simulink model "Base_Model_three_drones"  (R2025b)
settings: Solver=FixedStepDiscrete  StartTime=0.0  StopTime=10.0  FixedStep=0.01  RelTol=1e-3
values from neighbouring files (symbols this model uses):
  Attachment_Point_Vectors : value not decoded    [Base_Model.sldd]
  Cable_Damping = 0.1    [Base_Model.sldd]
  Cable_Resting_Length = 0.8    [Base_Model.sldd]
  Cable_Stiffness = 500.0    [Base_Model.sldd]
  Carrier_Mass = 0.01    [Base_Model.sldd]
  g = 9.81    [Base_Model.sldd]
  Kdc = 0.001    [Base_Model.sldd]
  Kpc = 10.0    [Base_Model.sldd]
  Load_Damping_Coef = 1.0    [Base_Model.sldd]
  Load_Inertia_Matrix : value not decoded    [Base_Model.sldd]
  Load_Mass = 0.7    [Base_Model.sldd]
undefined symbols (not defined in the file or in its folder): DiscIntNeverNeededParam
libraries: RotorSuite_lib x7, matrix_library x1, aerolibutil x1
settings Model: DataDictionary=Base_Model.sldd  Creator=lenovo  LastModifiedBy=lenovo

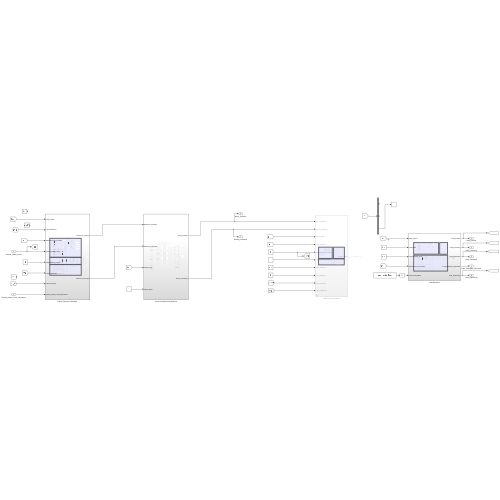
[thumbnail: Simulink's stored preview of the top-level diagram]
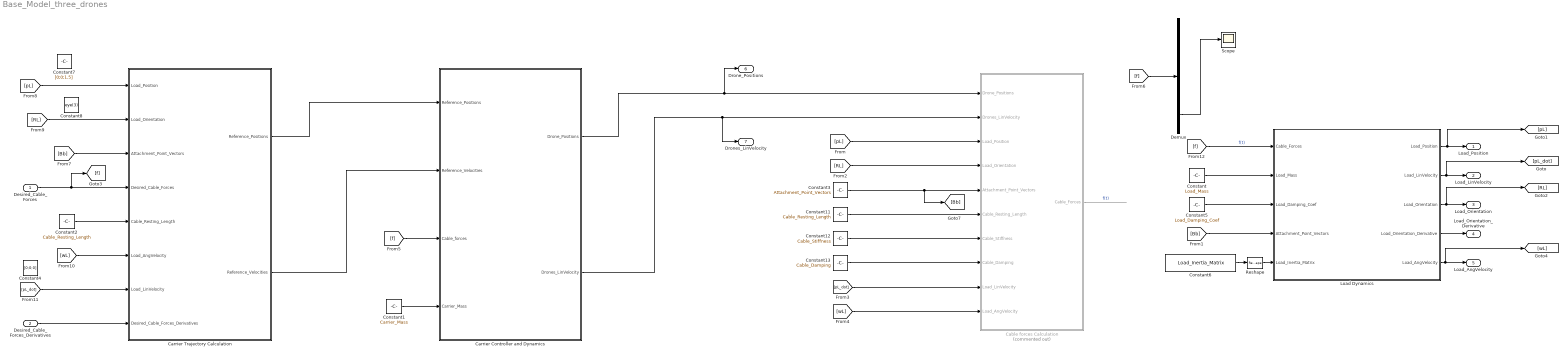
== system Base_Model_three_drones ==
  Desired_Cable_Forces : Inport
  Desired_Cable_Forces_Derivatives : Inport  Port=2
  Cable forces Calculation : Subsystem  Commented=on
  Carrier Controller and Dynamics : Subsystem
  "Carrier Trajectory Calculation " : Subsystem
  Constant : Constant  Value=Load_Mass
  Constant1 : Constant  Value=Carrier_Mass
  Constant11 : Constant  Value=Cable_Resting_Length
  Constant12 : Constant  Value=Cable_Stiffness
  Constant13 : Constant  Value=Cable_Damping
  Constant2 : Constant  Value=Cable_Resting_Length
  Constant3 : Constant  Value=Attachment_Point_Vectors
  Constant4 : Constant  Value=[0;0;0]
  Constant5 : Constant  Value=Load_Damping_Coef
  Constant6 : Constant  Value=Load_Inertia_Matrix
  Constant7 : Constant  Value=[0;0;1.5]
  Constant8 : Constant  Value=eye(3)
  Demux : Demux  Outputs=[3, 3, 3]
  Load Dynamics : Subsystem
  Reshape : Reshape  OutputDimensionality=Customize  OutputDimensions=[3,3]
  Scope : Scope
      settings: ActiveDisplayYMinimum=-1.9150350713046473E+13  ActiveDisplayYMaximum=2.47705516980144E+13
  Load_Position : Outport
  Load_LinVelocity : Outport  Port=2
  Load_Orientation : Outport  Port=3
  Load_Orientation_Derivative : Outport  Port=4
  Load_AngVelocity : Outport  Port=5
  Drone_Positions : Outport  Port=6
  Drones_LinVelocity : Outport  Port=7
  wires:
  Constant/1 -> Load Dynamics/2(Load_Mass)
  Constant5/1 -> Load Dynamics/3(Load_Damping_Coef)
  Constant6/1 -> Reshape/1
  Load Dynamics/2(Load_LinVelocity) -> [pL_dot], Load_LinVelocity/1
  Load Dynamics/1(Load_Position) -> [pL], Load_Position/1
  Load Dynamics/3(Load_Orientation) -> [RL], Load_Orientation/1
  Load Dynamics/5(Load_AngVelocity) -> [wL], Load_AngVelocity/1
  Cable forces Calculation/1(Cable_Forces) -> ?  "f(t)"
  [pL] -> Cable forces Calculation/3(Load_Position)
  [RL] -> Cable forces Calculation/4(Load_Orientation)
  Constant11/1 -> Cable forces Calculation/6(Cable_Resting_Length)
  [pL_dot] -> Cable forces Calculation/9(Load_LinVelocity)
  [wL] -> Cable forces Calculation/10(Load_AngVelocity)
  Constant12/1 -> Cable forces Calculation/7(Cable_Stiffness)
  Constant13/1 -> Cable forces Calculation/8(Cable_Damping)
  [Bb] -> Load Dynamics/4(Attachment_Point_Vectors)
  Carrier Controller and Dynamics/2(Drones_LinVelocity) -> Drones_LinVelocity/1, Cable forces Calculation/2(Drones_LinVelocity)
  [f] -> Carrier Controller and Dynamics/3(Cable_forces)
  Constant1/1 -> Carrier Controller and Dynamics/4(Carrier_Mass)
  "Carrier Trajectory Calculation "/1(Reference_Positions) -> Carrier Controller and Dynamics/1(Reference_Positions)
  Desired_Cable_Forces/1 -> [f], "Carrier Trajectory Calculation "/4(Desired_Cable_Forces)
  "Carrier Trajectory Calculation "/2(Reference_Velocities) -> Carrier Controller and Dynamics/2(Reference_Velocities)
  [Bb] -> "Carrier Trajectory Calculation "/3(Attachment_Point_Vectors)
  Constant2/1 -> "Carrier Trajectory Calculation "/5(Cable_Resting_Length)
  [wL] -> "Carrier Trajectory Calculation "/6(Load_AngVelocity)
  Desired_Cable_Forces_Derivatives/1 -> "Carrier Trajectory Calculation "/8(Desired_Cable_Forces_Derivatives)
  Load Dynamics/4(Load_Orientation_Derivative) -> Load_Orientation_Derivative/1
  Constant3/1 -> [Bb], Cable forces Calculation/5(Attachment_Point_Vectors)
  Reshape/1 -> Load Dynamics/5(Load_Inertia_Matrix)
  Demux/3 -> Scope/1
  [pL] -> "Carrier Trajectory Calculation "/1(Load_Position)
  [pL_dot] -> "Carrier Trajectory Calculation "/7(Load_LinVelocity)
  [f] -> Load Dynamics/1(Cable_Forces)  "f(t)"
  [f] -> Demux/1
  Carrier Controller and Dynamics/1(Drone_Positions) -> Drone_Positions/1, Cable forces Calculation/1(Drone_Positions)
  [RL] -> "Carrier Trajectory Calculation "/2(Load_Orientation)

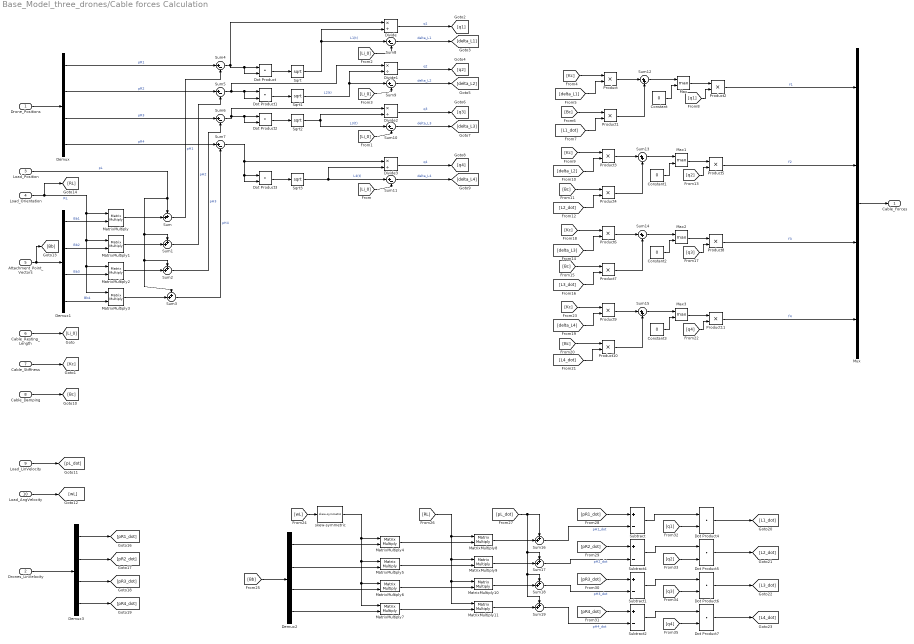
== system Base_Model_three_drones/Cable forces Calculation ==
  Drone_Positions : Inport
  Drones_LinVelocity : Inport  Port=2
  Load_Position : Inport  Port=3
  Load_Orientation : Inport  Port=4
  Attachment_Point_Vectors : Inport  Port=5
  Cable_Resting_Length : Inport  Port=6
  Cable_Stiffness : Inport  Port=7
  Cable_Damping : Inport  Port=8
  Load_LinVelocity : Inport  Port=9
  Load_AngVelocity : Inport  Port=10
  Constant{,1..3} (4 alike) : Constant  Value=0
  Demux : Demux
  Demux1 : Demux  Outputs=[3, 3, 3, 3]
  Demux2 : Demux
  Demux3 : Demux
  Divide{,1..3} (4 alike) : Product  Inputs=*/
  Dot Product{,1..7} (8 alike) : DotProduct  OutDataTypeStr=Inherit: Inherit via internal rule
  MatrixMultiply{,1..11} (12 alike) : Product  Multiplication=Matrix(*)
  Max{,1..3} (4 alike) : MinMax  Function=max  Inputs=2
  Mux : Mux
  Product{,1..11} (12 alike) : Product
  Sqrt{,1..3} (4 alike) : Sqrt
  Subtract{,1..2,4} (4 alike) : Sum  Inputs=+-
  Sum{,1..3,16..19} (8 alike) : Sum  Inputs=++|
  Sum{4..11} (8 alike) : Sum  Inputs=|+-
  Sum{12..15} (4 alike) : Sum  Inputs=|++
  skew-symmetric : RotorSuite_lib/Utils/skew-symmetric
  Cable_Forces : Outport
  wires:
  Mux/1 -> Cable_Forces/1
  Drone_Positions/1 -> Demux/1
  Attachment_Point_Vectors/1 -> Demux1/1, [Bb]
  Demux1/1 -> MatrixMultiply/2  "Bb1"
  Load_Orientation/1 -> [RL], MatrixMultiply3/1, MatrixMultiply2/1, MatrixMultiply1/1, MatrixMultiply/1  "RL"
  Demux1/2 -> MatrixMultiply1/2  "Bb2"
  Demux1/3 -> MatrixMultiply2/2  "Bb3"
  Demux1/4 -> MatrixMultiply3/2  "Bb4"
  MatrixMultiply/1 -> Sum/2
  Load_Position/1 -> Sum1/1, Sum2/1, Sum3/1, Sum/1  "pL"
  MatrixMultiply1/1 -> Sum1/2
  MatrixMultiply2/1 -> Sum2/2
  MatrixMultiply3/1 -> Sum3/2
  Demux/1 -> Sum4/1  "pR1"
  Demux/2 -> Sum5/1  "pR2"
  Demux/3 -> Sum6/1  "pR3"
  Demux/4 -> Sum7/1  "pR4"
  Sum/1 -> Sum4/2  "pH1"
  Sum1/1 -> Sum5/2  "pH2"
  Sum2/1 -> Sum6/2  "pH3"
  Sum3/1 -> Sum7/2  "pH4"
  Sum4/1 -> Dot Product/2, Dot Product/1, Divide/1
  Dot Product/1 -> Sqrt/1
  Dot Product1/1 -> Sqrt1/1
  Dot Product2/1 -> Sqrt2/1
  Dot Product3/1 -> Sqrt3/1
  Sqrt/1 -> Divide/2, Sum8/1  "L1(t)"
  Sqrt1/1 -> Sum9/1, Divide1/2  "L2(t)"
  Sum5/1 -> Dot Product1/2, Dot Product1/1, Divide1/1
  Sqrt2/1 -> Sum10/1, Divide2/2  "L3(t)"
  Sum6/1 -> Divide2/1, Dot Product2/2, Dot Product2/1
  Sqrt3/1 -> Divide3/2, Sum11/1  "L4(t)"
  Sum7/1 -> Divide3/1, Dot Product3/2, Dot Product3/1
  Cable_Resting_Length/1 -> [Li_0]
  Cable_Stiffness/1 -> [Kc]
  [Li_0] -> Sum11/2
  [Li_0] -> Sum10/2
  [Li_0] -> Sum8/2
  [Li_0] -> Sum9/2
  Divide/1 -> [q1]  "q1"
  Divide1/1 -> [q2]  "q2"
  Divide2/1 -> [q3]  "q3"
  Divide3/1 -> [q4]  "q4"
  Sum8/1 -> [delta_L1]  "delta_L1"
  Sum9/1 -> [delta_L2]  "delta_L2"
  Sum10/1 -> [delta_L3]  "delta_L3"
  Sum11/1 -> [delta_L4]  "delta_L4"
  [Kc] -> Product/1
  [delta_L1] -> Product/2
  Cable_Damping/1 -> [Bc]
  [L1_dot] -> Product1/2
  [Bc] -> Product1/1
  Product/1 -> Sum12/1
  Product1/1 -> Sum12/2
  Sum12/1 -> Max/1
  Constant/1 -> Max/2
  Max/1 -> Product2/1
  [q1] -> Product2/2
  Product2/1 -> Mux/1  "f1"
  [q2] -> Product5/2
  Max1/1 -> Product5/1
  Constant1/1 -> Max1/2
  Sum13/1 -> Max1/1
  Product4/1 -> Sum13/2
  Product3/1 -> Sum13/1
  [Bc] -> Product4/1
  [L2_dot] -> Product4/2
  [delta_L2] -> Product3/2
  [Kc] -> Product3/1
  Product5/1 -> Mux/2  "f2"
  [Kc] -> Product6/1
  [delta_L3] -> Product6/2
  [L3_dot] -> Product7/2
  [Bc] -> Product7/1
  Product6/1 -> Sum14/1
  Product7/1 -> Sum14/2
  Sum14/1 -> Max2/1
  Constant2/1 -> Max2/2
  Max2/1 -> Product8/1
  [q3] -> Product8/2
  Product8/1 -> Mux/3  "f3"
  [q4] -> Product11/2
  Max3/1 -> Product11/1
  Constant3/1 -> Max3/2
  Sum15/1 -> Max3/1
  Product10/1 -> Sum15/2
  Product9/1 -> Sum15/1
  [Bc] -> Product10/1
  [L4_dot] -> Product10/2
  [delta_L4] -> Product9/2
  [Kc] -> Product9/1
  Product11/1 -> Mux/4  "f4"
  Load_LinVelocity/1 -> [pL_dot]
  Load_AngVelocity/1 -> [wL]
  [Bb] -> Demux2/1
  [wL] -> skew-symmetric/1
  Demux2/1 -> MatrixMultiply4/2
  Demux2/2 -> MatrixMultiply5/2
  Demux2/3 -> MatrixMultiply6/2
  Demux2/4 -> MatrixMultiply7/2
  skew-symmetric/1 -> MatrixMultiply5/1, MatrixMultiply6/1, MatrixMultiply7/1, MatrixMultiply4/1
  MatrixMultiply4/1 -> MatrixMultiply8/2
  MatrixMultiply5/1 -> MatrixMultiply9/2
  MatrixMultiply6/1 -> MatrixMultiply10/2
  MatrixMultiply7/1 -> MatrixMultiply11/2
  [RL] -> MatrixMultiply11/1, MatrixMultiply10/1, MatrixMultiply9/1, MatrixMultiply8/1
  MatrixMultiply8/1 -> Sum16/2
  MatrixMultiply9/1 -> Sum17/2
  MatrixMultiply10/1 -> Sum18/2
  MatrixMultiply11/1 -> Sum19/2
  [pL_dot] -> Sum16/1, Sum19/1, Sum18/1, Sum17/1
  Drones_LinVelocity/1 -> Demux3/1
  Demux3/1 -> [pR1_dot]
  Demux3/2 -> [pR2_dot]
  Demux3/3 -> [pR3_dot]
  Demux3/4 -> [pR4_dot]
  Sum16/1 -> Subtract/2  "pH1_dot"
  [pR1_dot] -> Subtract/1
  [pR2_dot] -> Subtract4/1
  Sum17/1 -> Subtract4/2  "pH2_dot"
  [pR3_dot] -> Subtract1/1
  Sum18/1 -> Subtract1/2  "pH3_dot"
  Sum19/1 -> Subtract2/2  "pH4_dot"
  [pR4_dot] -> Subtract2/1
  Subtract/1 -> Dot Product4/1
  [q1] -> Dot Product4/2
  Subtract4/1 -> Dot Product5/1
  Subtract1/1 -> Dot Product6/1
  Subtract2/1 -> Dot Product7/1
  [q2] -> Dot Product5/2
  [q3] -> Dot Product6/2
  [q4] -> Dot Product7/2
  Dot Product4/1 -> [L1_dot]
  Dot Product5/1 -> [L2_dot]
  Dot Product6/1 -> [L3_dot]
  Dot Product7/1 -> [L4_dot]

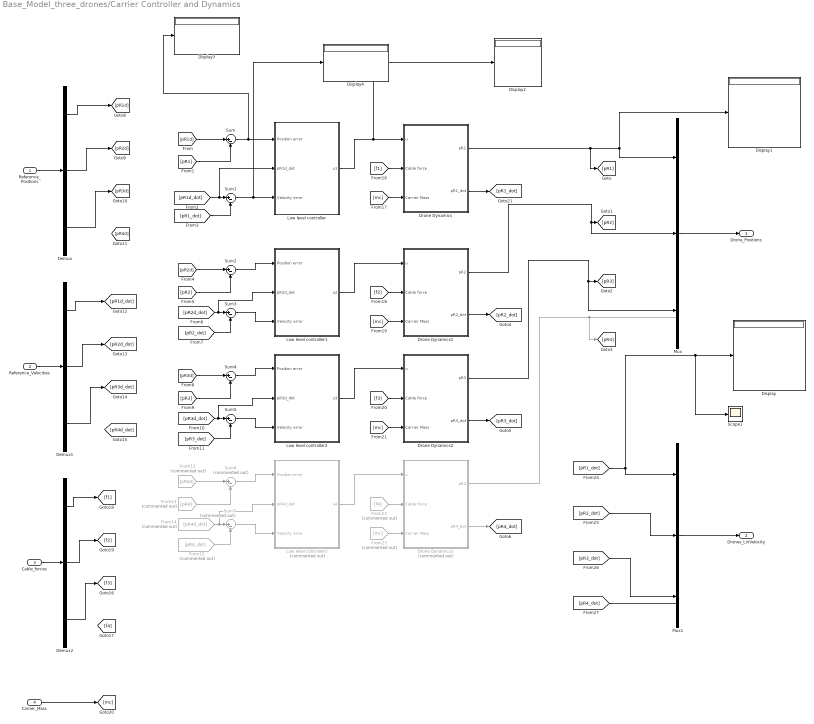
== system Base_Model_three_drones/Carrier Controller and Dynamics ==
  Reference_Positions : Inport
  Reference_Velocities : Inport  Port=2
  Cable_forces : Inport  Port=3
  Carrier_Mass : Inport  Port=4
  Demux : Demux  Outputs=3
  Demux1 : Demux  Outputs=3
  Demux2 : Demux  Outputs=3
  Display{,1..4} (5 alike) : Display
  Drone Dynamics : Subsystem
  Drone Dynamics1 : Subsystem
  Drone Dynamics2 : Subsystem
  Drone Dynamics3 : Subsystem  Commented=on
  From12 : From  Commented=on  GotoTag=pR4d
  From13 : From  Commented=on  GotoTag=pR4
  From14 : From  Commented=on  GotoTag=pR4d_dot
  From15 : From  Commented=on  GotoTag=pR4_dot
  From22 : From  Commented=on  GotoTag=f4
  From23 : From  Commented=on  GotoTag=mc
  Low level controller : Subsystem
  Low level controller1 : Subsystem
  Low level controller2 : Subsystem
  Low level controller3 : Subsystem  Commented=on
  Mux : Mux  Inputs=3
  Mux1 : Mux  Inputs=3
  Scope1 : Scope
      settings: ActiveDisplayYMinimum=-1  ActiveDisplayYMaximum=1  DataLoggingVariableName=ScopeData2
  Sum{,1..5} (6 alike) : Sum  Inputs=|+-
  Sum6 : Sum  Commented=on  Inputs=|+-
  Sum7 : Sum  Commented=on  Inputs=|+-
  Drone_Positions : Outport
  Drones_LinVelocity : Outport  Port=2
  wires:
  Mux/1 -> Drone_Positions/1
  Mux1/1 -> Drones_LinVelocity/1
  Reference_Positions/1 -> Demux/1
  Reference_Velocities/1 -> Demux1/1
  Drone Dynamics2/1(pR3) -> [pR3], Mux/3
  Drone Dynamics3/1(pR4) -> [pR4]
  Drone Dynamics1/1(pR2) -> [pR2], Mux/2
  [pR3_dot] -> Mux1/3
  [pR2_dot] -> Mux1/2
  [pR1_dot] -> Scope1/1, Display/1, Mux1/1
  [pR4_dot] -> ?
  Demux/1 -> [pR1d]
  Demux/2 -> [pR2d]
  Demux/3 -> [pR3d]
  ? -> [pR4d]
  Demux1/1 -> [pR1d_dot]
  Demux1/2 -> [pR2d_dot]
  Demux1/3 -> [pR3d_dot]
  ? -> [pR4d_dot]
  [pR1d] -> Sum/1
  [pR1] -> Sum/2
  Sum/1 -> Display3/1, Low level controller/1(Position error)
  [pR1_dot] -> Sum1/2
  [pR1d_dot] -> Low level controller/2(pR1d_dot), Sum1/1
  Sum1/1 -> Display4/1, Low level controller/3(Velocity error)
  [pR2d_dot] -> Low level controller1/2(pR2d_dot), Sum3/1
  [pR2_dot] -> Sum3/2
  [pR2] -> Sum2/2
  Sum2/1 -> Low level controller1/1(Position error)
  Sum3/1 -> Low level controller1/3(Velocity error)
  [pR2d] -> Sum2/1
  [pR3] -> Sum4/2
  [pR3d_dot] -> Low level controller2/2(pR3d_dot), Sum5/1
  [pR3d] -> Sum4/1
  From12/1 -> Sum6/1
  Sum5/1 -> Low level controller2/3(Velocity error)
  Sum6/1 -> Low level controller3/1(Position error)
  [pR3_dot] -> Sum5/2
  From13/1 -> Sum6/2
  From15/1 -> Sum7/2
  Sum7/1 -> Low level controller3/3(Velocity error)
  From14/1 -> Low level controller3/2(pR4d_dot), Sum7/1
  Sum4/1 -> Low level controller2/1(Position error)
  Cable_forces/1 -> Demux2/1
  Demux2/1 -> [f1]
  Demux2/2 -> [f2]
  Demux2/3 -> [f3]
  ? -> [f4]
  Carrier_Mass/1 -> [mc]
  [f1] -> Drone Dynamics/2(Cable force)
  [mc] -> Drone Dynamics/3(Carrier Mass)
  Low level controller1/1(u2) -> Drone Dynamics1/1(u)
  [f2] -> Drone Dynamics1/2(Cable force)
  [mc] -> Drone Dynamics1/3(Carrier Mass)
  [mc] -> Drone Dynamics2/3(Carrier Mass)
  [f3] -> Drone Dynamics2/2(Cable force)
  Low level controller2/1(u3) -> Drone Dynamics2/1(u)
  Low level controller3/1(u4) -> Drone Dynamics3/1(u)
  From23/1 -> Drone Dynamics3/3(Carrier Mass)
  From22/1 -> Drone Dynamics3/2(Cable force)
  Drone Dynamics/2(pR1_dot) -> [pR1_dot]
  Drone Dynamics1/2(pR2_dot) -> [pR2_dot]
  Drone Dynamics2/2(pR3_dot) -> [pR3_dot]
  Drone Dynamics3/2(pR4_dot) -> [pR4_dot]
  Low level controller/1(u1) -> Display2/1, Drone Dynamics/1(u)
  Drone Dynamics/1(pR1) -> [pR1], Display1/1, Mux/1

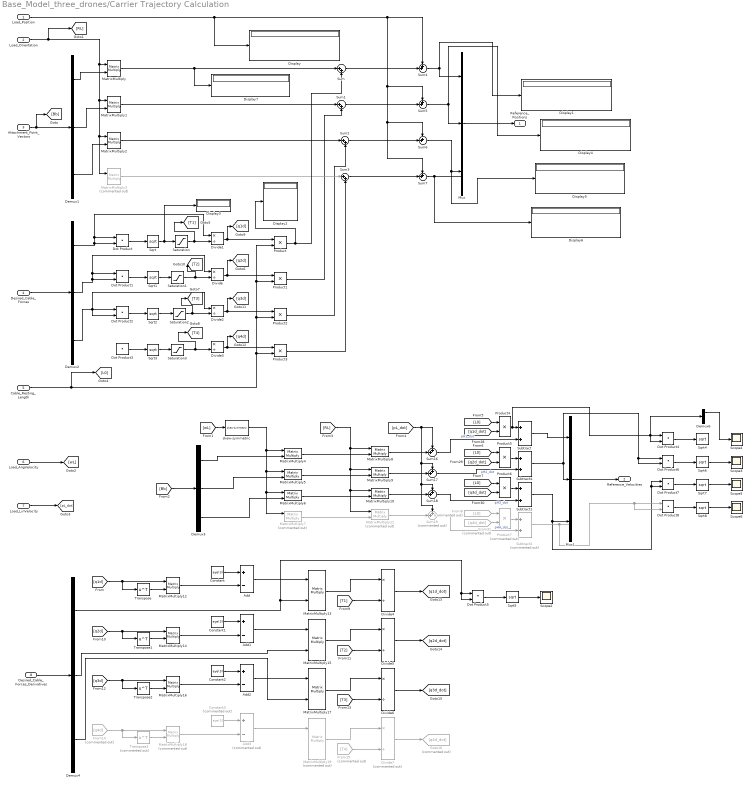
== system Base_Model_three_drones/Carrier Trajectory Calculation  ==
  Load_Position : Inport
  Load_Orientation : Inport  Port=2
  Attachment_Point_Vectors : Inport  Port=3
  Desired_Cable_Forces : Inport  Port=4
  Cable_Resting_Length : Inport  Port=5
  Load_AngVelocity : Inport  Port=6
  Load_LinVelocity : Inport  Port=7
  Desired_Cable_Forces_Derivatives : Inport  Port=8
  Add : Sum  Inputs=+-
  Add1 : Sum  Inputs=+-
  Add2 : Sum  Inputs=+-
  Add3 : Sum  Commented=on  Inputs=+-
  Constant : Constant  Value=eye(3)
  Constant1 : Constant  Value=eye(3)
  Constant2 : Constant  Value=eye(3)
  Constant3 : Constant  Commented=on  Value=eye(3)
  Demux{1..4} (4 alike) : Demux  Outputs=[3, 3, 3]
  Demux6 : Demux  Outputs=3
  Display{,1..7} (8 alike) : Display
  Divide{,1..6} (7 alike) : Product  Inputs=*/
  Divide7 : Product  Commented=on  Inputs=*/
  Dot Product{,1..8} (9 alike) : DotProduct  OutDataTypeStr=Inherit: Inherit via internal rule
  From14 : From  Commented=on  GotoTag=q4d
  From15 : From  Commented=on  GotoTag=T4
  From31 : From  Commented=on  GotoTag=q4d_dot
  From8 : From  Commented=on  GotoTag=L0
  Goto16 : Goto  Commented=on  GotoTag=q4d_dot
  MatrixMultiply{,1..2,4..6,8..10,12..17} (15 alike) : Product  Multiplication=Matrix(*)
  MatrixMultiply{3,7,11,18..19} (5 alike) : Product  Commented=on  Multiplication=Matrix(*)
  Mux : Mux  Inputs=3
  Mux1 : Mux  Inputs=3
  Product{,1..6} (7 alike) : Product
  Product7 : Product  Commented=on
  Saturation{,1..3} (4 alike) : Saturate  UpperLimit=inf  LowerLimit=0.00001
  Scope{2..6} (5 alike) : Scope
      Scope2 settings: ActiveDisplayYMinimum=-4.0782199553181471  ActiveDisplayYMaximum=26.499977935087504  DataLoggingVariableName=ScopeData3
      Scope3 settings: ActiveDisplayYMinimum=-0.80772325667978673  ActiveDisplayYMaximum=7.2695093101180825  DataLoggingVariableName=ScopeData4
      Scope4 settings: ActiveDisplayYMinimum=-0.0816381655658385  ActiveDisplayYMaximum=0.73474349009254614
      Scope5 settings: ActiveDisplayYMinimum=-0.16312920034811029  ActiveDisplayYMaximum=1.468162803132993  DataLoggingVariableName=ScopeData6
      Scope6 settings: ActiveDisplayYMinimum=-0.16312920034811029  ActiveDisplayYMaximum=1.468162803132993  DataLoggingVariableName=ScopeData7
  Sqrt{,1..8} (9 alike) : Sqrt
  Subtract : Sum
  Subtract1 : Sum
  Subtract2 : Sum  Commented=on
  Subtract4 : Sum
  Sum{,1..3} (4 alike) : Sum  Inputs=|++
  Sum{4..7,16..18} (7 alike) : Sum  Inputs=++|
  Sum19 : Sum  Commented=on  Inputs=++|
  Transpose : Math  Operator=transpose
  Transpose1 : Math  Operator=transpose
  Transpose2 : Math  Operator=transpose
  Transpose3 : Math  Commented=on  Operator=transpose
  skew-symmetric : RotorSuite_lib/Utils/skew-symmetric
  Reference_Positions : Outport
  Reference_Velocities : Outport  Port=2
  wires:
  Desired_Cable_Forces/1 -> Demux2/1
  ? -> MatrixMultiply3/2
  Demux1/3 -> MatrixMultiply2/2
  Demux1/2 -> MatrixMultiply1/2
  Demux1/1 -> MatrixMultiply/2
  Attachment_Point_Vectors/1 -> [Bb], Demux1/1
  Mux1/1 -> Reference_Velocities/1
  Mux/1 -> Reference_Positions/1
  Load_Orientation/1 -> [RL], MatrixMultiply3/1, MatrixMultiply2/1, MatrixMultiply1/1, MatrixMultiply/1
  Dot Product/1 -> Sqrt/1
  Dot Product1/1 -> Sqrt1/1
  Demux2/2 -> Divide/1, Dot Product1/1, Dot Product1/2
  Dot Product2/1 -> Sqrt2/1
  Demux2/3 -> Dot Product2/2, Divide2/1, Dot Product2/1
  ? -> Dot Product3/2, Divide3/1, Dot Product3/1
  Dot Product3/1 -> Sqrt3/1
  Sqrt/1 -> Display3/1, Saturation/1
  Sqrt2/1 -> Saturation2/1
  Sqrt3/1 -> Saturation3/1
  Cable_Resting_Length/1 -> [L0], Product3/2, Product2/2, Product1/2, Product/2
  MatrixMultiply1/1 -> Sum1/1
  Product1/1 -> Sum1/2
  MatrixMultiply2/1 -> Sum2/1
  Product2/1 -> Sum2/2
  MatrixMultiply3/1 -> Sum3/1
  Product3/1 -> Sum3/2
  Load_Position/1 -> Display/1, Sum4/1, Sum6/1, Sum7/1, Sum5/1
  MatrixMultiply/1 -> Display7/1, Sum/1
  Product/1 -> Display2/1, Sum/2
  Sum/1 -> Sum4/2
  Sum1/1 -> Sum5/2
  Sum2/1 -> Sum6/2
  Sum3/1 -> Sum7/2
  Sum4/1 -> Display1/1, Mux/1
  Sum5/1 -> Display4/1, Mux/2
  Sum6/1 -> Display5/1, Mux/3
  Sum7/1 -> Display6/1
  MatrixMultiply6/1 -> MatrixMultiply10/2
  MatrixMultiply5/1 -> MatrixMultiply9/2
  skew-symmetric/1 -> MatrixMultiply5/1, MatrixMultiply6/1, MatrixMultiply7/1, MatrixMultiply4/1
  Demux3/2 -> MatrixMultiply5/2
  MatrixMultiply11/1 -> Sum19/2
  [wL] -> skew-symmetric/1
  MatrixMultiply4/1 -> MatrixMultiply8/2
  [Bb] -> Demux3/1
  MatrixMultiply10/1 -> Sum18/2
  [q3d_dot] -> Product6/2
  MatrixMultiply9/1 -> Sum17/2
  [pL_dot] -> Sum16/1, Sum19/1, Sum18/1, Sum17/1
  Demux3/1 -> MatrixMultiply4/2
  MatrixMultiply7/1 -> MatrixMultiply11/2
  [RL] -> MatrixMultiply11/1, MatrixMultiply10/1, MatrixMultiply9/1, MatrixMultiply8/1
  ? -> MatrixMultiply7/2
  MatrixMultiply8/1 -> Sum16/2
  Demux3/3 -> MatrixMultiply6/2
  Load_AngVelocity/1 -> [wL]
  Load_LinVelocity/1 -> [pL_dot]
  [q1d_dot] -> Product4/2
  [L0] -> Product4/1
  [L0] -> Product5/1
  Product5/1 -> Subtract4/1
  [q2d_dot] -> Product5/2
  [L0] -> Product6/1
  Product6/1 -> Subtract1/1
  From8/1 -> Product7/1
  Product7/1 -> Subtract2/1
  From31/1 -> Product7/2
  Subtract/1 -> Mux1/1
  Subtract1/1 -> Dot Product7/1, Dot Product7/2, Mux1/3
  Subtract2/1 -> Dot Product8/2, Dot Product8/1
  Desired_Cable_Forces_Derivatives/1 -> Demux4/1
  Sqrt1/1 -> Saturation1/1
  Demux2/1 -> Divide1/1, Dot Product/1, Dot Product/2
  Divide/1 -> Product1/1, [q2d]
  Divide1/1 -> [q1d], Product/1
  Divide2/1 -> [q3d], Product2/1
  Divide3/1 -> Product3/1, [q4d]
  Constant/1 -> Add/1
  [q1d] -> MatrixMultiply12/1, Transpose/1
  MatrixMultiply12/1 -> Add/2
  Transpose/1 -> MatrixMultiply12/2
  Add/1 -> MatrixMultiply13/1
  Demux4/1 -> Dot Product5/2, Dot Product5/1, MatrixMultiply13/2
  MatrixMultiply13/1 -> Divide4/1
  [T1] -> Divide4/2
  Divide5/1 -> [q2d_dot]
  Constant1/1 -> Add1/1
  MatrixMultiply14/1 -> Add1/2
  [q2d] -> MatrixMultiply14/1, Transpose1/1
  Add1/1 -> MatrixMultiply15/1
  MatrixMultiply15/1 -> Divide5/1
  Transpose1/1 -> MatrixMultiply14/2
  Demux4/2 -> MatrixMultiply15/2
  [T2] -> Divide5/2
  Divide6/1 -> [q3d_dot]
  Constant2/1 -> Add2/1
  MatrixMultiply16/1 -> Add2/2
  [q3d] -> MatrixMultiply16/1, Transpose2/1
  Add2/1 -> MatrixMultiply17/1
  MatrixMultiply17/1 -> Divide6/1
  Transpose2/1 -> MatrixMultiply16/2
  Demux4/3 -> MatrixMultiply17/2
  [T3] -> Divide6/2
  Divide7/1 -> Goto16/1
  Constant3/1 -> Add3/1
  MatrixMultiply18/1 -> Add3/2
  From14/1 -> MatrixMultiply18/1, Transpose3/1
  Add3/1 -> MatrixMultiply19/1
  MatrixMultiply19/1 -> Divide7/1
  Transpose3/1 -> MatrixMultiply18/2
  ? -> MatrixMultiply19/2
  From15/1 -> Divide7/2
  Saturation/1 -> [T1], Divide1/2
  Saturation1/1 -> Divide/2, [T2]
  Saturation2/1 -> [T3], Divide2/2
  Saturation3/1 -> [T4], Divide3/2
  Subtract4/1 -> Dot Product6/2, Dot Product6/1, Mux1/2
  Dot Product4/1 -> Sqrt4/1
  Divide4/1 -> [q1d_dot]
  Dot Product5/1 -> Sqrt5/1
  Dot Product6/1 -> Sqrt6/1
  Sqrt6/1 -> Scope3/1
  Sqrt7/1 -> Scope5/1
  Dot Product7/1 -> Sqrt7/1
  Dot Product8/1 -> Sqrt8/1
  Sqrt8/1 -> Scope6/1
  Sqrt5/1 -> Scope2/1
  Product4/1 -> Demux6/1, Dot Product4/2, Dot Product4/1, Subtract/1
  Sum16/1 -> Subtract/2  "pH1_dot"
  Sum17/1 -> Subtract4/2  "pH2_dot"
  Sum18/1 -> Subtract1/2  "pH3_dot"
  Sum19/1 -> Subtract2/2  "pH4_dot"
  Demux6/1 -> Scope4/1

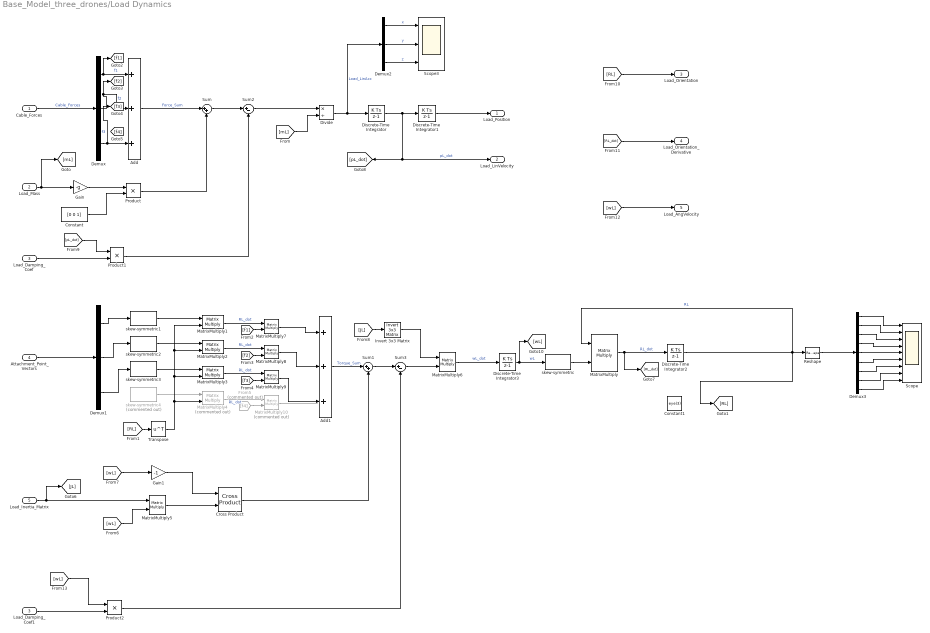
== system Base_Model_three_drones/Load Dynamics ==
  Cable_Forces : Inport
  Load_Mass : Inport  Port=2
  Load_Damping_Coef : Inport  Port=3
  Attachment_Point_Vectors : Inport  Description=Attachment Point Vectors in body frame  Port=4
  Load_Inertia_Matrix : Inport  Port=5
  Add : Sum  Inputs=+++
  Add1 : Sum  Inputs=+++
  Constant : Constant  Value=[0 0 1]
  Constant1 : Constant  Value=eye(3)
  Cross Product : matrix_library/Cross Product
  Demux : Demux  Outputs=[3, 3, 3]
  Demux1 : Demux  Outputs=[3, 3, 3]
  Demux2 : Demux  Outputs=3
  Demux3 : Demux  Outputs=9
  Discrete-Time Integrator : DiscreteIntegrator  SampleTime=-1  ICPrevOutput=DiscIntNeverNeededParam  ICPrevScaledInput=DiscIntNeverNeededParam
  Discrete-Time Integrator1 : DiscreteIntegrator  InitialCondition=[0; 0; 1.4]  SampleTime=-1  ICPrevOutput=DiscIntNeverNeededParam  ICPrevScaledInput=DiscIntNeverNeededParam
  Discrete-Time Integrator2 : DiscreteIntegrator  InitialCondition=eye(3)  SampleTime=-1  ICPrevOutput=DiscIntNeverNeededParam  ICPrevScaledInput=DiscIntNeverNeededParam
  Discrete-Time Integrator3 : DiscreteIntegrator  SampleTime=-1  ICPrevOutput=DiscIntNeverNeededParam  ICPrevScaledInput=DiscIntNeverNeededParam
  Divide : Product  Inputs=*/
  From5 : From  Commented=on  GotoTag=f4
  Gain : Gain  Gain=-g
  Gain1 : Gain  Gain=-1
  Invert 3x3 Matrix : aerolibutil/Invert  3x3 Matrix
  Load_Damping_Coef1 : InportShadow  Port=3
  MatrixMultiply{,1..3,5..9} (9 alike) : Product  Multiplication=Matrix(*)
  MatrixMultiply10 : Product  Commented=on  Multiplication=Matrix(*)
  MatrixMultiply4 : Product  Commented=on  Multiplication=Matrix(*)
  Product : Product
  Product1 : Product
  Product2 : Product
  Reshape : Reshape
  Scope : Scope  NumInputPorts=9
      settings: ActiveDisplayYMinimum=0.9  ActiveDisplayYMaximum=1.1  DataLoggingVariableName=ScopeData8
  Scope3 : Scope  NumInputPorts=3
      settings: ActiveDisplayYMinimum=-9.802338570910781E-14  ActiveDisplayYMaximum=8.8221047138197057E-13  DataLoggingVariableName=Load_x2
  Sum : Sum  Inputs=|++
  Sum1 : Sum  Inputs=|++
  Sum2 : Sum  Inputs=|+-
  Sum3 : Sum  Inputs=|+-
  Transpose : Math  Operator=transpose
  skew-symmetric{,1..3} (4 alike) : RotorSuite_lib/Utils/skew-symmetric
  skew-symmetric4 : RotorSuite_lib/Utils/skew-symmetric  Commented=on
  Load_Position : Outport
  Load_LinVelocity : Outport  Port=2
  Load_Orientation : Outport  Port=3
  Load_Orientation_Derivative : Outport  Port=4
  Load_AngVelocity : Outport  Port=5
  wires:
  Cable_Forces/1 -> Demux/1  "Cable_Forces"
  Demux/1 -> [f1], Add/1  "f1"
  Demux/2 -> Add/2, [f2]  "f2"
  Demux/3 -> [f3], Add/3  "f3"
  ? -> [f4]  "f4"
  Load_Mass/1 -> [mL], Gain/1
  Gain/1 -> Product/1
  Constant/1 -> Product/2
  Add/1 -> Sum/1  "Force_Sum"
  Product/1 -> Sum/2
  [mL] -> Divide/2
  Discrete-Time Integrator/1 -> Discrete-Time Integrator1/1, Load_LinVelocity/1, [pL_dot]  "pL_dot"
  Discrete-Time Integrator1/1 -> Load_Position/1
  skew-symmetric/1 -> MatrixMultiply/2
  MatrixMultiply/1 -> [RL_dot], Discrete-Time Integrator2/1  "RL_dot"
  [RL] -> Transpose/1
  Attachment_Point_Vectors/1 -> Demux1/1
  Demux1/1 -> skew-symmetric1/1
  Demux1/2 -> skew-symmetric2/1
  Demux1/3 -> skew-symmetric3/1
  ? -> skew-symmetric4/1
  skew-symmetric1/1 -> MatrixMultiply1/1
  skew-symmetric2/1 -> MatrixMultiply2/1
  skew-symmetric3/1 -> MatrixMultiply3/1
  skew-symmetric4/1 -> MatrixMultiply4/1
  Transpose/1 -> MatrixMultiply1/2, MatrixMultiply2/2, MatrixMultiply3/2, MatrixMultiply4/2
  MatrixMultiply7/1 -> Add1/1
  MatrixMultiply8/1 -> Add1/2
  MatrixMultiply9/1 -> Add1/3
  MatrixMultiply10/1 -> ?
  Add1/1 -> Sum1/1  "Torque_Sum"
  Load_Inertia_Matrix/1 -> [JL], MatrixMultiply5/1
  [wL] -> MatrixMultiply5/2
  MatrixMultiply5/1 -> Cross Product/2
  [wL] -> Gain1/1
  Gain1/1 -> Cross Product/1
  Cross Product/1 -> Sum1/2
  [JL] -> Invert 3x3 Matrix/1
  Invert 3x3 Matrix/1 -> MatrixMultiply6/1
  MatrixMultiply6/1 -> Discrete-Time Integrator3/1  "wL_dot"
  Discrete-Time Integrator3/1 -> skew-symmetric/1, [wL]  "wL"
  [f1] -> MatrixMultiply7/2
  MatrixMultiply1/1 -> MatrixMultiply7/1  "RL_dot"
  MatrixMultiply2/1 -> MatrixMultiply8/1  "RL_dot"
  [f2] -> MatrixMultiply8/2
  MatrixMultiply3/1 -> MatrixMultiply9/1  "RL_dot"
  [f3] -> MatrixMultiply9/2
  MatrixMultiply4/1 -> MatrixMultiply10/1  "RL_dot"
  From5/1 -> MatrixMultiply10/2
  [RL] -> Load_Orientation/1
  [wL] -> Load_AngVelocity/1
  Sum/1 -> Sum2/1
  Sum2/1 -> Divide/1
  [pL_dot] -> Product1/1
  Load_Damping_Coef/1 -> Product1/2
  [RL_dot] -> Load_Orientation_Derivative/1
  Load_Damping_Coef1/1 -> Product2/2
  [wL] -> Product2/1
  Sum1/1 -> Sum3/1
  Sum3/1 -> MatrixMultiply6/2
  Product2/1 -> Sum3/2
  Divide/1 -> Demux2/1, Discrete-Time Integrator/1  "Load_LinAcc"
  Demux2/2 -> Scope3/2  "y"
  Demux2/1 -> Scope3/1  "x"
  Demux2/3 -> Scope3/3  "z"
  Product1/1 -> Sum2/2
  Discrete-Time Integrator2/1 -> [RL], MatrixMultiply/1, Reshape/1  "RL"
  Demux3/6 -> Scope/6
  Demux3/8 -> Scope/8
  Demux3/7 -> Scope/7
  Demux3/9 -> Scope/9
  Reshape/1 -> Demux3/1
  Demux3/2 -> Scope/2
  Demux3/3 -> Scope/3
  Demux3/1 -> Scope/1
  Demux3/4 -> Scope/4
  Demux3/5 -> Scope/5

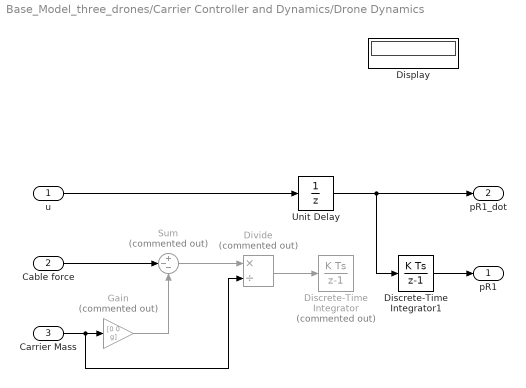
== system Base_Model_three_drones/Carrier Controller and Dynamics/Drone Dynamics ==
  u : Inport
  Cable force : Inport  Port=2
  Carrier Mass : Inport  Port=3
  Discrete-Time Integrator : DiscreteIntegrator  Commented=on  SampleTime=-1  ICPrevOutput=DiscIntNeverNeededParam  ICPrevScaledInput=DiscIntNeverNeededParam
  Discrete-Time Integrator1 : DiscreteIntegrator  InitialCondition=[1;1;2.3]  SampleTime=-1  ICPrevOutput=DiscIntNeverNeededParam  ICPrevScaledInput=DiscIntNeverNeededParam
  Display : Display
  Divide : Product  Commented=on  Inputs=*/
  Gain : Gain  Commented=on  Gain=[0 0 g]
  Sum : Sum  Commented=on  Inputs=+--
  Unit Delay : UnitDelay  SampleTime=-1  HasFrameUpgradeWarning=on
  pR1 : Outport
  pR1_dot : Outport  Port=2
  wires:
  Cable force/1 -> Sum/2
  Carrier Mass/1 -> Divide/2, Gain/1
  Gain/1 -> Sum/3
  Sum/1 -> Divide/1
  Divide/1 -> Discrete-Time Integrator/1
  Discrete-Time Integrator1/1 -> pR1/1
  u/1 -> Unit Delay/1
  Unit Delay/1 -> pR1_dot/1, Discrete-Time Integrator1/1

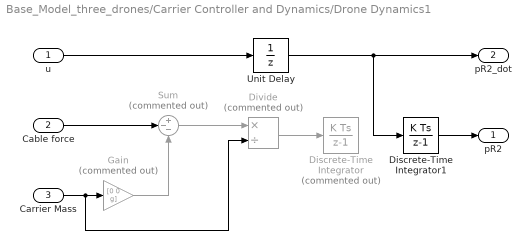
== system Base_Model_three_drones/Carrier Controller and Dynamics/Drone Dynamics1 ==
  u : Inport
  Cable force : Inport  Port=2
  Carrier Mass : Inport  Port=3
  Discrete-Time Integrator : DiscreteIntegrator  Commented=on  SampleTime=-1  ICPrevOutput=DiscIntNeverNeededParam  ICPrevScaledInput=DiscIntNeverNeededParam
  Discrete-Time Integrator1 : DiscreteIntegrator  InitialCondition=[-1;1;2.3]  SampleTime=-1  ICPrevOutput=DiscIntNeverNeededParam  ICPrevScaledInput=DiscIntNeverNeededParam
  Divide : Product  Commented=on  Inputs=*/
  Gain : Gain  Commented=on  Gain=[0 0 g]
  Sum : Sum  Commented=on  Inputs=+--
  Unit Delay : UnitDelay  SampleTime=-1  HasFrameUpgradeWarning=on
  pR2 : Outport
  pR2_dot : Outport  Port=2
  wires:
  Cable force/1 -> Sum/2
  Carrier Mass/1 -> Divide/2, Gain/1
  Gain/1 -> Sum/3
  Divide/1 -> Discrete-Time Integrator/1
  Discrete-Time Integrator1/1 -> pR2/1
  Sum/1 -> Divide/1
  u/1 -> Unit Delay/1
  Unit Delay/1 -> Discrete-Time Integrator1/1, pR2_dot/1

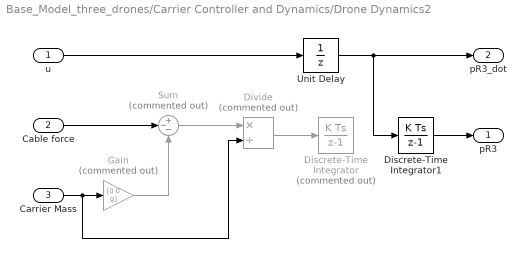
== system Base_Model_three_drones/Carrier Controller and Dynamics/Drone Dynamics2 ==
  u : Inport
  Cable force : Inport  Port=2
  Carrier Mass : Inport  Port=3
  Discrete-Time Integrator : DiscreteIntegrator  Commented=on  SampleTime=-1  ICPrevOutput=DiscIntNeverNeededParam  ICPrevScaledInput=DiscIntNeverNeededParam
  Discrete-Time Integrator1 : DiscreteIntegrator  InitialCondition=[-1;-1;2.3]  SampleTime=-1  ICPrevOutput=DiscIntNeverNeededParam  ICPrevScaledInput=DiscIntNeverNeededParam
  Divide : Product  Commented=on  Inputs=*/
  Gain : Gain  Commented=on  Gain=[0 0 g]
  Sum : Sum  Commented=on  Inputs=+--
  Unit Delay : UnitDelay  SampleTime=-1  HasFrameUpgradeWarning=on
  pR3 : Outport
  pR3_dot : Outport  Port=2
  wires:
  Cable force/1 -> Sum/2
  Carrier Mass/1 -> Gain/1, Divide/2
  Gain/1 -> Sum/3
  Sum/1 -> Divide/1
  Divide/1 -> Discrete-Time Integrator/1
  Discrete-Time Integrator1/1 -> pR3/1
  u/1 -> Unit Delay/1
  Unit Delay/1 -> Discrete-Time Integrator1/1, pR3_dot/1

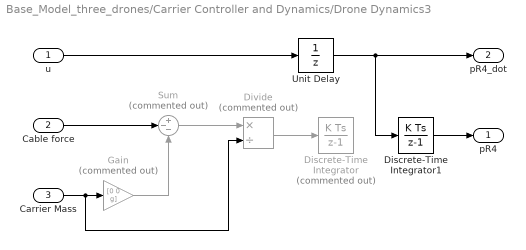
== system Base_Model_three_drones/Carrier Controller and Dynamics/Drone Dynamics3 ==
  u : Inport
  Cable force : Inport  Port=2
  Carrier Mass : Inport  Port=3
  Discrete-Time Integrator : DiscreteIntegrator  Commented=on  SampleTime=-1  ICPrevOutput=DiscIntNeverNeededParam  ICPrevScaledInput=DiscIntNeverNeededParam
  Discrete-Time Integrator1 : DiscreteIntegrator  InitialCondition=[1;-1;2.3]  SampleTime=-1  ICPrevOutput=DiscIntNeverNeededParam  ICPrevScaledInput=DiscIntNeverNeededParam
  Divide : Product  Commented=on  Inputs=*/
  Gain : Gain  Commented=on  Gain=[0 0 g]
  Sum : Sum  Commented=on  Inputs=+--
  Unit Delay : UnitDelay  SampleTime=-1  HasFrameUpgradeWarning=on
  pR4 : Outport
  pR4_dot : Outport  Port=2
  wires:
  Sum/1 -> Divide/1
  Gain/1 -> Sum/3
  Carrier Mass/1 -> Divide/2, Gain/1
  Cable force/1 -> Sum/2
  Discrete-Time Integrator1/1 -> pR4/1
  Divide/1 -> Discrete-Time Integrator/1
  u/1 -> Unit Delay/1
  Unit Delay/1 -> Discrete-Time Integrator1/1, pR4_dot/1

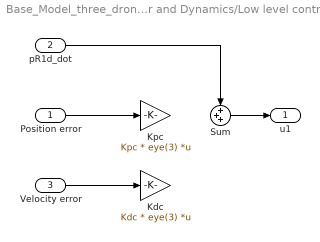
== system Base_Model_three_drones/Carrier Controller and Dynamics/Low level controller ==
  Position error : Inport
  pR1d_dot : Inport  Port=2
  Velocity error : Inport  Port=3
  Kdc : Gain  Gain=Kdc * eye(3)  Multiplication=Matrix(K*u) (u vector)
  Kpc : Gain  Gain=Kpc * eye(3)  Multiplication=Matrix(K*u) (u vector)
  Sum : Sum  Inputs=+++
  u1 : Outport
  wires:
  Position error/1 -> Kpc/1
  Velocity error/1 -> Kdc/1
  Sum/1 -> u1/1
  pR1d_dot/1 -> Sum/1

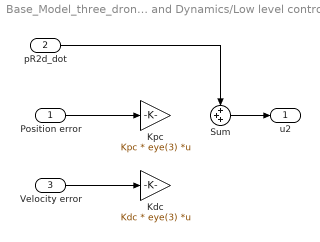
== system Base_Model_three_drones/Carrier Controller and Dynamics/Low level controller1 ==
  Position error : Inport
  pR2d_dot : Inport  Port=2
  Velocity error : Inport  Port=3
  Kdc : Gain  Gain=Kdc * eye(3)  Multiplication=Matrix(K*u) (u vector)
  Kpc : Gain  Gain=Kpc * eye(3)  Multiplication=Matrix(K*u) (u vector)
  Sum : Sum  Inputs=+++
  u2 : Outport
  wires:
  Position error/1 -> Kpc/1
  Velocity error/1 -> Kdc/1
  Sum/1 -> u2/1
  pR2d_dot/1 -> Sum/1

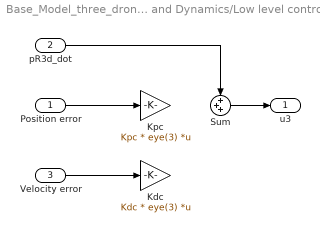
== system Base_Model_three_drones/Carrier Controller and Dynamics/Low level controller2 ==
  Position error : Inport
  pR3d_dot : Inport  Port=2
  Velocity error : Inport  Port=3
  Kdc : Gain  Gain=Kdc * eye(3)  Multiplication=Matrix(K*u) (u vector)
  Kpc : Gain  Gain=Kpc * eye(3)  Multiplication=Matrix(K*u) (u vector)
  Sum : Sum  Inputs=+++
  u3 : Outport
  wires:
  Position error/1 -> Kpc/1
  Velocity error/1 -> Kdc/1
  Sum/1 -> u3/1
  pR3d_dot/1 -> Sum/1

== system Base_Model_three_drones/Carrier Controller and Dynamics/Low level controller3 ==
  Position error : Inport
  pR4d_dot : Inport  Port=2
  Velocity error : Inport  Port=3
  Kdc : Gain  Gain=Kdc * eye(3)  Multiplication=Matrix(K*u) (u vector)
  Kpc : Gain  Gain=Kpc * eye(3)  Multiplication=Matrix(K*u) (u vector)
  Sum : Sum  Inputs=+++
  u4 : Outport
  wires:
  Position error/1 -> Kpc/1
  Velocity error/1 -> Kdc/1
  Sum/1 -> u4/1
  pR4d_dot/1 -> Sum/1
